simulink model "vertical"  (R2025a)
settings: Solver=VariableStepAuto  StartTime=0.0  StopTime=10.0  RelTol=1e-3
InitFcn:
  | vehicleData = readJson(simConfig.vehicleConfigFile);
model workspace (MAT data in the model file):
  Param = Simulink.Parameter
  Param.Complexity = 'real'
  Param.Dimensions = [0 0]
  Param.DataType = 'auto'
settings Model: Creator=marce  LastModifiedBy=marce

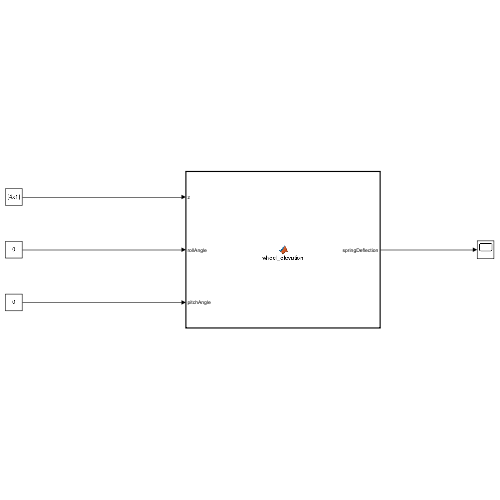
[thumbnail: Simulink's stored preview of the top-level diagram]
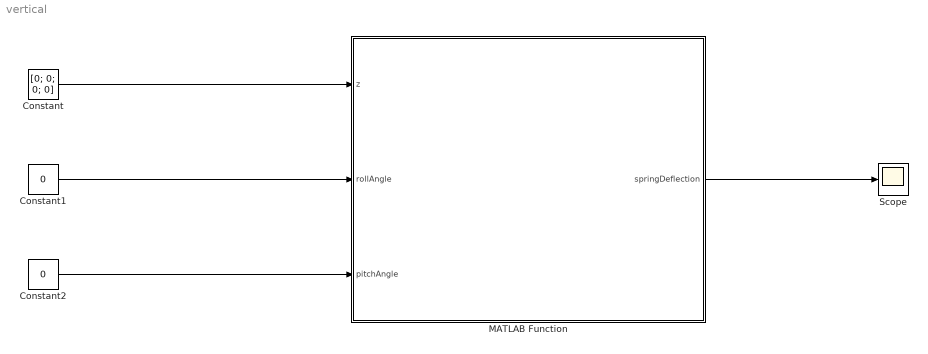
== system vertical ==
  Constant : Constant  Value=[0; 0; 0; 0]
  Constant1 : Constant  Value=0
  Constant2 : Constant  Value=0
  MATLAB Function : MATLAB Function  TreatAsAtomicUnit=on
  Scope : Scope
  wires:
  Constant/1 -> MATLAB Function/1(z)
  Constant1/1 -> MATLAB Function/2(rollAngle)
  Constant2/1 -> MATLAB Function/3(pitchAngle)
  MATLAB Function/1(springDeflection) -> Scope/1

== matlab function vertical/MATLAB Function ==
  data: z input; rollAngle input; springDeflection output; pitchAngle input; vehicleData data_store_memory
function springDeflection = wheel_elevation(z, rollAngle, pitchAngle)

l = vehicleData.dimensions.wheelbase_mm;
lnzv = vehicleData.vertical_parameters.distance_to_pitch_center_front_mm;
sv = vehicleData.dimensions.track_width_front_mm;
sh = vehicleData.dimensions.track_width_rear_mm;

c = 0.5 * (-1).^[1:4]';

trackMultipliers = [sv; sv; sh; sh];
pitchMultipliers = [lnzv; lnzv; (l-lnzv); (l-lnzv)];

springDeflection = z .* ones(4,1) ...
                   + sin(rollAngle) .* (c .* trackMultipliers) ...
                   + sin(pitchAngle) .* pitchMultipliers;
